simulink model "step5_observor_test"  (R2021b)
settings: Solver=FixedStepAuto  StartTime=0.0  StopTime=RunTime  FixedStep=time_step  RelTol=1e-3
values from neighbouring files (symbols this model uses):
  A = [0 1 0 0 ... (first row only)    [linearize_script.m]    (also in step4_0_linearize_operating_point.m = double(A); step4_linearized_system.mat = [0 0.339319496362 0 -114.426616159 0 1 -102.612245897 0 221.; syms_test.m = double(A))
  B = [0 ... (first row only)    [linearize_script.m]    (also in step4_0_linearize_operating_point.m = double(B); step4_linearized_system.mat = [0 0 0 0 5076.90787281]; syms_test.m = double(B))
  C = [1 0 0 0 ... (first row only)    [linearize_script.m]    (also in matrixmaker_linearization.m = [b_1_0 - P_3 * theta_d_2 * sin(theta_2)  -P_3 * (theta_d_1 +; step4_0_linearize_operating_point.m = [1 0 0 0 0; step4_linearized_system.mat = [1  0  0  0  0; 0  0  1  0  0]; syms_test.m)
  D = zeros(2,1)    [linearize_script.m]    (also in step4_0_linearize_operating_point.m; step4_linearized_system.mat = [0 0]; syms_test.m)
  g1 = (m_1 * c_1_0 + m_2 * l_1) * g    [compare_ourmodel_with_others.m]    (also in step2_whitebox_beam.m; step4_0_linearize_operating_point.m = (m1 * c1 + m2 * l1) * g; step5_observor_design.m = (m1 * c1 + m2 * l1) * g; step6_1_controller_feedback.m)
  g2 = m_2 * c_2_0 * g    [compare_ourmodel_with_others.m]    (also in step2_whitebox_beam.m; step4_0_linearize_operating_point.m = m2 * c2 * g; step5_observor_design.m = m2 * c2 * g; step6_1_controller_feedback.m)
  Ke = [165.387583111  -5.89857635124; 3165.93278733  -398.274578992; 81.102554045  215.74157361; 15046.5760039  11054.3649817; 3886.10400765  -704.144825536]    [step5_observor.mat]    (also in step5_observor_design.m = place(A_, B_, 0.5*J)')
  P1 = m_1 * c_1_0 * c_1_0 + m_2 * l_1 * l_1 + I_1_0    [compare_ourmodel_with_others.m]    (also in script_for_test.m = P2(1:L/2+1); step2_whitebox_beam.m; step4_0_linearize_operating_point.m = m1 * c1 * c1 + m2 * l1 * l1 + I1; step5_observor_design.m = m1 * c1 * c1 + m2 * l1 * l1 + I1)
  P2 = m_2 * c_2_0 * c_2_0 + I_2_0    [compare_ourmodel_with_others.m]    (also in script_for_test.m = abs(Y/L); step2_whitebox_beam.m; step4_0_linearize_operating_point.m = m2 * c2 * c2 + I2; step5_observor_design.m = m2 * c2 * c2 + I2)
  P3 = m_2 * l_1 * c_2_0    [compare_ourmodel_with_others.m]    (also in step2_whitebox_beam.m; step4_0_linearize_operating_point.m = m2 * l1 * c2; step5_observor_design.m = m2 * l1 * c2; step6_1_controller_feedback.m)
  params = [9.81, 0.1, 0.1, 0.125, 0.05, -0.1, 0.040, 0.054196, 0.0001744, 5.6468, 1.57151198693013e-05, 18.9174724265491, 0.000501346852070284]    [compare_ourmodel_with_others.m]    (also in linearization.m = params_hat; matrixmaker_linearization.m = [-0.001, 0.077, 0.2, 0.00004, 20.684, 0.0004, 15, 0.03]; params.mat = [9.81 0.1 0.1 0.125 0.046955 -0.032 0.04609 0.0888 9.9e-05 6; sss.m = [9.81, 0.1, 0.1, 0.125, 0.04824, -0.041443, .0607558, 0.1154)
  theta_1_0 = pi    (= 3.14159265359)    [hwinit.m]    (also in hwinit_raw.m; step4_0_linearize_operating_point.m; step5_observor_design.m = x_op(1); step6_1_controller_feedback.m = x_op(1))
  theta_2_0 = 0    [hwinit.m]    (also in hwinit_raw.m; step4_0_linearize_operating_point.m; step5_observor_design.m = x_op(3); step6_1_controller_feedback.m = x_op(3))
  x_op_relative = [0; 0; 0; 0; 0]    [step5_observor_design.m]    (also in step6_1_controller_feedback.m)
settings Model: Creator=annel  LastModifiedBy=97083
settings DebuggingCC: UnconnectedInputMsg=none  UnconnectedOutputMsg=none  UnconnectedLineMsg=none
settings ModelReferenceCC: EnableRefExpFcnMdlSchedulingChecks=off
settings RTWCC: DLArmComputeVersion=20.02.1

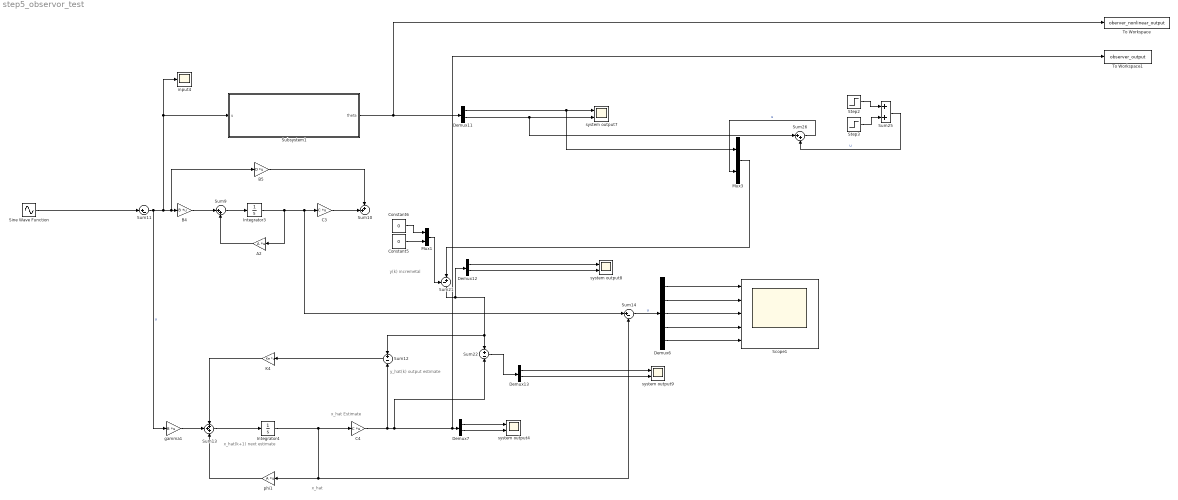
== system step5_observor_test ==
  note: y_hat(k)
      | output estimate
  note: x_hat
  note: y(k)
      | incremetal
  note: x_hat(k+1)
      | next estimate
  note: x_hat
      | Estimate
  A2 : Gain  Gain=A  Multiplication=Matrix(K*u) (u vector)
  B4 : Gain  Gain=B  Multiplication=Matrix(K*u)
  B5 : Gain  Gain=D  Multiplication=Matrix(K*u)
  C3 : Gain  Gain=C  Multiplication=Matrix(K*u) (u vector)
  C4 : Gain  Gain=C  Multiplication=Matrix(K*u) (u vector)
  Constant5 : Constant  Value=0  SampleTime=-1
  Constant6 : Constant  Value=0  SampleTime=-1
  Demux{7,11..13} (4 alike) : Demux  Outputs=2
  Demux6 : Demux  Outputs=5
  Integrator3 : Integrator  InitialCondition=x_op_relative
  Integrator4 : Integrator  InitialCondition=x_op_relative
  K4 : Gain  Gain=Ke  Multiplication=Matrix(K*u) (u vector)
  Mux1 : Mux  Inputs=2
  Mux3 : Mux  Inputs=2
  Scope1 : Scope  NumInputPorts=5
  Sine Wave Function : Sin  Amplitude=0.05  Frequency=2*pi*2  SampleTime=0.001
  Step2 : Step  After=0.1  SampleTime=0
  Step3 : Step  Time=1.05  After=-0.1  SampleTime=0
  Subsystem1 : Subsystem
  Sum10 : Sum  Inputs=++|
  Sum11 : Sum  Inputs=|+-
  Sum12 : Sum  Inputs=+|-
  Sum13 : Sum  Inputs=+++
  Sum14 : Sum  Inputs=|+-
  Sum21 : Sum  Inputs=-+|
  Sum22 : Sum  Inputs=+|-
  Sum25 : Sum
  Sum26 : Sum  Inputs=|++
  Sum9 : Sum  Inputs=|++
  To Workspace : ToWorkspace  VariableName=oberver_nonlinear_output  SampleTime=0.001
  To Workspace1 : ToWorkspace  VariableName=observer_output  SampleTime=0.001
  gamma1 : Gain  Gain=B  Multiplication=Matrix(K*u)
  input4 : Scope
  phi1 : Gain  Gain=A  Multiplication=Matrix(K*u) (u vector)
  system output{4,7..9} (4 alike) : Scope  NumInputPorts=2
  wires:
  Demux6/5 -> Scope1/5
  Demux6/4 -> Scope1/4
  Demux6/3 -> Scope1/3
  Demux6/2 -> Scope1/2
  Demux6/1 -> Scope1/1
  Demux7/1 -> system output4/1
  Demux7/2 -> system output4/2
  C4/1 -> Sum12/2, Sum22/2, To Workspace1/1, Demux7/1
  Sum14/1 -> Demux6/1  "u"
  phi1/1 -> Sum13/3
  Sum12/1 -> K4/1
  Sum13/1 -> Integrator4/1
  K4/1 -> Sum13/1
  gamma1/1 -> Sum13/2
  Integrator4/1 -> phi1/1, Sum14/2, C4/1
  A2/1 -> Sum9/2
  B4/1 -> Sum9/1
  Sum11/1 -> Subsystem1/1(u), input4/1, B4/1, B5/1, gamma1/1  "u"
  Sum9/1 -> Integrator3/1
  Sine Wave Function/1 -> Sum11/1
  C3/1 -> Sum10/2
  Integrator3/1 -> C3/1, Sum14/1, A2/1
  B5/1 -> Sum10/1
  Constant6/1 -> Mux1/1
  Constant5/1 -> Mux1/2
  Mux1/1 -> Sum21/1
  Sum21/1 -> Sum12/1, Sum22/1, Demux12/1
  Demux12/1 -> system output8/1
  Demux12/2 -> system output8/2
  Sum22/1 -> Demux13/1
  Demux13/2 -> system output9/2
  Demux13/1 -> system output9/1
  Demux11/2 -> Sum26/1, system output7/2
  Sum26/1 -> Mux3/2  "u"
  Sum25/1 -> Sum26/2  "u"
  Step2/1 -> Sum25/1
  Demux11/1 -> Mux3/1, system output7/1
  Step3/1 -> Sum25/2
  Mux3/1 -> Sum21/2
  Subsystem1/1(theta) -> To Workspace/1, Demux11/1

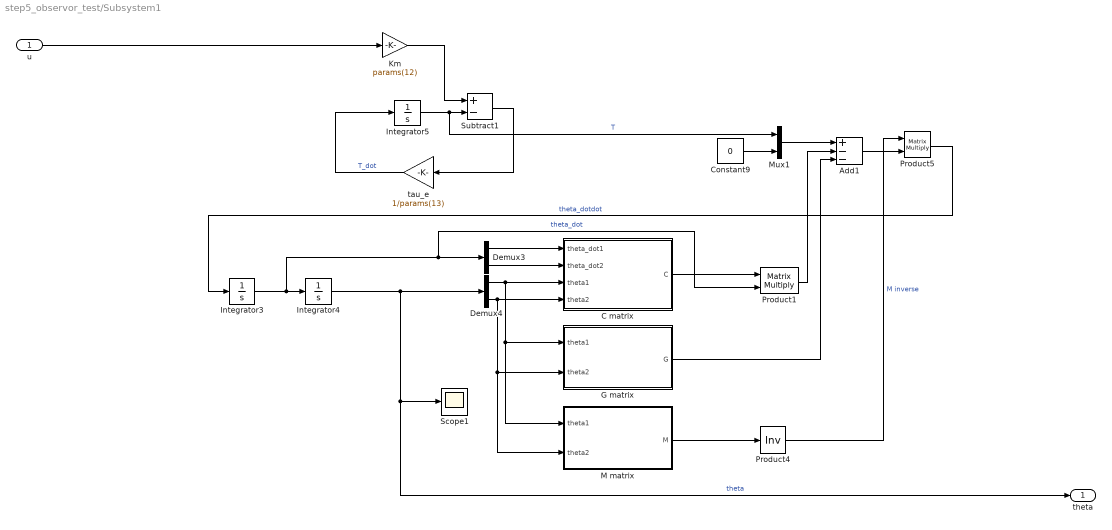
== system step5_observor_test/Subsystem1 ==
  u : Inport
  Add1 : Sum  Inputs=+--
  C matrix : MATLAB Function  TreatAsAtomicUnit=on
  Constant9 : Constant  Value=0
  Demux3 : Demux  Outputs=2
  Demux4 : Demux  Outputs=2
  G matrix : MATLAB Function  TreatAsAtomicUnit=on
  Integrator3 : Integrator
  Integrator4 : Integrator  InitialCondition=[theta_1_0 theta_2_0]
  Integrator5 : Integrator
  Km : Gain  Gain=params(12)
  M matrix : MATLAB Function  TreatAsAtomicUnit=on
  Mux1 : Mux  Inputs=2
  Product1 : Product  Inputs=**  Multiplication=Matrix(*)
  Product4 : Product  Inputs=/  Multiplication=Matrix(*)
  Product5 : Product  Inputs=**  Multiplication=Matrix(*)
  Scope1 : Scope
  Subtract1 : Sum  Inputs=+-
  tau_e : Gain  Gain=1/params(13)
  theta : Outport
  wires:
  Demux4/1 -> M matrix/1(theta1), G matrix/1(theta1), C matrix/3(theta1)
  tau_e/1 -> Integrator5/1  "T_dot"
  Constant9/1 -> Mux1/2
  Demux3/1 -> C matrix/1(theta_dot1)
  Add1/1 -> Product5/2
  Subtract1/1 -> tau_e/1
  G matrix/1(G) -> Add1/3
  Integrator3/1 -> Product1/2, Demux3/1, Integrator4/1  "theta_dot"
  C matrix/1(C) -> Product1/1
  Mux1/1 -> Add1/1
  Integrator5/1 -> Mux1/1, Subtract1/2  "T"
  u/1 -> Km/1
  Product5/1 -> Integrator3/1  "theta_dotdot"
  Demux3/2 -> C matrix/2(theta_dot2)
  Integrator4/1 -> Demux4/1, theta/1, Scope1/1  "theta"
  M matrix/1(M) -> Product4/1
  Demux4/2 -> M matrix/2(theta2), G matrix/2(theta2), C matrix/4(theta2)
  Product4/1 -> Product5/1  "M inverse"
  Product1/1 -> Add1/2
  Km/1 -> Subtract1/1

== matlab function step5_observor_test/Subsystem1/C matrix ==
  data: theta_dot1 input; theta_dot2 input; theta1 input; theta2 input; C output; params parameter; P3 parameter
function C = C(theta_dot1, theta_dot2, theta1, theta2, params, P3)
c00 = params(10) - P3 * theta_dot2 * sin(theta2);
c01 = -P3 * (theta_dot1 + theta_dot2) * sin(theta2);
c10 = P3 * theta_dot1 * sin(theta2);
c11 = params(11);

C = [c00 c01;
     c10 c11];

== matlab function step5_observor_test/Subsystem1/G matrix ==
  data: theta1 input; theta2 input; G output; g1 parameter; g2 parameter
function G = G(theta1, theta2, g1, g2)
G00 = -g1 * sin(theta1) - g2 * sin(theta1 + theta2);
G01 = -g2 * sin(theta1 + theta2);

G = [G00 G01];

== matlab function step5_observor_test/Subsystem1/M matrix ==
  data: theta1 input; theta2 input; M output; P1 parameter; P2 parameter; P3 parameter
function M = fcn(theta1, theta2, P1, P2, P3)
M00 = P1 + P2 + 2 * P3 * cos(theta2);
M01 = P2 + P3 * cos(theta2);
M10 = M01;
M11 = P2;

M = [M00 M01;
     M10 M11];
